simulink model "A1trim"  (R2018a)
settings: Solver=VariableStepAuto  StartTime=0.0  StopTime=10.0  RelTol=1e-3
model workspace (MATLAB code in the model file):
  | M = 20
  | a = 0.5
  | zf = 0.1
  | x10 = 0
  | x20 = 0
settings Model: Creator=Raj  LastModifiedBy=Raj

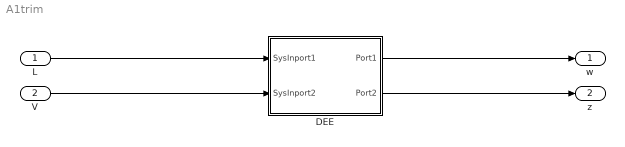
== system A1trim ==
  L : Inport
  V : Inport  Port=2
  DEE : Subsystem  mask(Differential Equation Editor (DEE)){}
      settings: OpenFcn=diffeqed
      mask Display: disp('Differential Equation\n Editor')
  w : Outport
  z : Outport  Port=2
  wires:
  L/1 -> DEE/1(SysInport1)
  V/1 -> DEE/2(SysInport2)
  DEE/1(Port1) -> w/1
  DEE/2(Port2) -> z/1

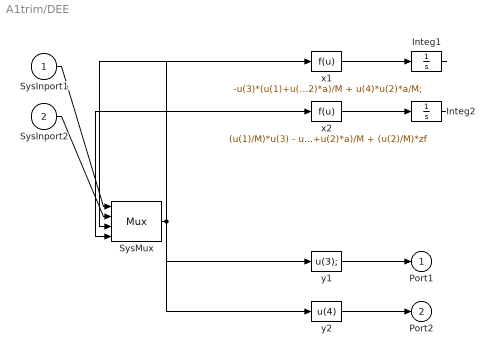
== system A1trim/DEE ==
  SysInport1 : Inport
  SysInport2 : Inport  Port=2
  Integ1 : Integrator  InitialCondition=x10
  Integ2 : Integrator  InitialCondition=x20
  SysMux : Mux
  x1 : Fcn  Expr=-u(3)*(u(1)+u(2)*a)/M + u(4)*u(2)*a/M;
  x2 : Fcn  Expr=(u(1)/M)*u(3) - u(4)*(u(1)+u(2)*a)/M + (u(2)/M)*zf
  y1 : Fcn  Expr=u(3);
  y2 : Fcn  Expr=u(4)
  Port1 : Outport
  Port2 : Outport  Port=2
  wires:
  SysInport1/1 -> SysMux/1
  SysInport2/1 -> SysMux/2
  SysMux/1 -> x1/1, x2/1, y1/1, y2/1
  x1/1 -> Integ1/1
  Integ1/1 -> SysMux/3
  x2/1 -> Integ2/1
  Integ2/1 -> SysMux/4
  y1/1 -> Port1/1
  y2/1 -> Port2/1
